simulink model "continuos_system"  (R2013a)
settings: Solver=ode45  StartTime=0.0  StopTime=10.0  RelTol=1e-3
settings Model: Creator=root  LastModifiedBy=root

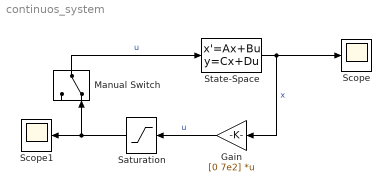
== system continuos_system ==
  Gain : Gain  Gain=[0 7e2]  Multiplication=Matrix(K*u)
  Manual Switch : ManualSwitch  CurrentSetting=0
  Saturation : Saturate  UpperLimit=150  LowerLimit=-150
  Scope : Scope
      settings: TimeRange=10
  Scope1 : Scope
      settings: TimeRange=10
  State-Space : StateSpace  A=[0 1; -(19.5^2) -2*19.5*0.01]  B=[0; 1e-4]  C=[1 0]  D=0  X0=[-2e-3; 0]
  wires:
  State-Space/1 -> Gain/1, Scope/1  "x"
  Manual Switch/1 -> State-Space/1  "u"
  Gain/1 -> Saturation/1  "u"
  Saturation/1 -> Scope1/1, Manual Switch/2
